simulink model "MBD_Mux_Demux"  (R2021b)
settings: Solver=FixedStepDiscrete  StartTime=0.0  StopTime=10.0  FixedStep=0.01  RelTol=1e-3
libraries: simulink x6
settings Model: Creator=waleed.elshemy  LastModifiedBy=waleed.elshemy

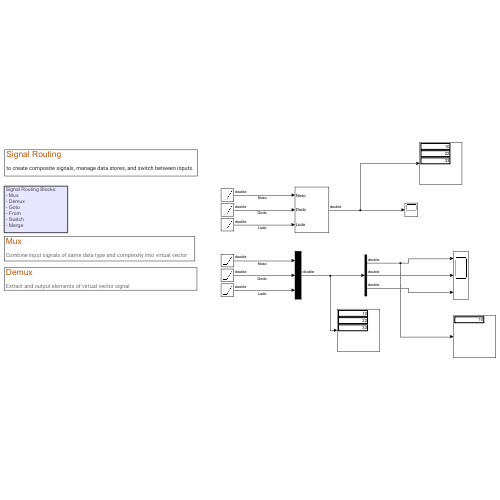
[thumbnail: Simulink's stored preview of the top-level diagram]
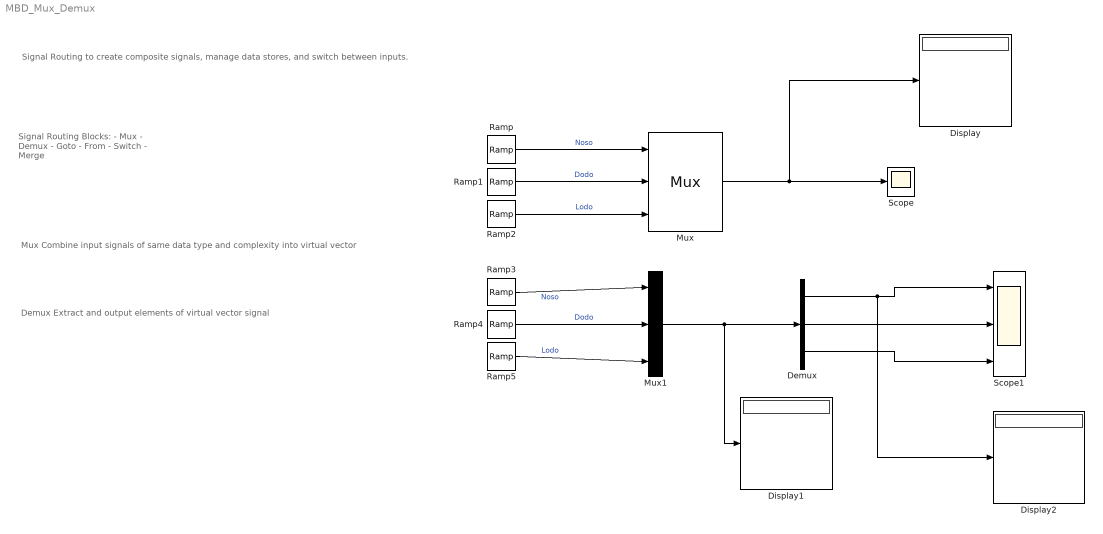
== system MBD_Mux_Demux ==
  note: Demux
      | Extract and output elements of virtual vector signal
  note: Signal Routing
      | to create composite signals, manage data stores, and switch between inputs.
  note: Signal Routing Blocks:
      | - Mux
      | - Demux
      | - Goto
      | - From
      | - Switch
      | - Merge
  note: Mux
      | Combine input signals of same data type and complexity into virtual vector
  Demux : Demux  Outputs=3
  Display : Display
  Display1 : Display
  Display2 : Display
  Mux : Mux  Inputs=3
      settings: DisplayOption=signals
  Mux1 : Mux  Inputs=3
  Ramp : simulink/Sources/Ramp  slope=1  start=0  InitialOutput=0
  Ramp1 : simulink/Sources/Ramp  slope=2  start=0  InitialOutput=2
  Ramp2 : simulink/Sources/Ramp  slope=3  start=0  InitialOutput=3
  Ramp3 : simulink/Sources/Ramp  slope=1  start=0  InitialOutput=0
  Ramp4 : simulink/Sources/Ramp  slope=2  start=0  InitialOutput=2
  Ramp5 : simulink/Sources/Ramp  slope=3  start=0  InitialOutput=3
  Scope : Scope
  Scope1 : Scope  NumInputPorts=3
  wires:
  Ramp/1 -> Mux/1  "Noso"
  Ramp1/1 -> Mux/2  "Dodo"
  Ramp2/1 -> Mux/3  "Lodo"
  Mux/1 -> Display/1, Scope/1
  Ramp5/1 -> Mux1/3  "Lodo"
  Ramp4/1 -> Mux1/2  "Dodo"
  Ramp3/1 -> Mux1/1  "Noso"
  Mux1/1 -> Display1/1, Demux/1
  Demux/1 -> Display2/1, Scope1/1
  Demux/2 -> Scope1/2
  Demux/3 -> Scope1/3
